simulink model "CubeSatTEST"  (R2024b)
settings: Solver=ode4  StartTime=simul.t0  StopTime=simul.tf  FixedStep=0.01  RelTol=1e-3
values from neighbouring files (symbols this model uses):
  alpha1 = 0.7    [mainSimTEST.m]
  alpha2 = 0.3    [mainSimTEST.m]
undefined symbols (not defined in the file or in its folder): act, DiscIntNeverNeededParam, env, flag, IC, K, orb, sat, sens
libraries: matrix_library x55, simulink_extras x5, simulink x2
(part 1 of 10)
settings Model: SimulationMode=accelerator  Creator=filippocamaleonte  LastModifiedBy=esteb

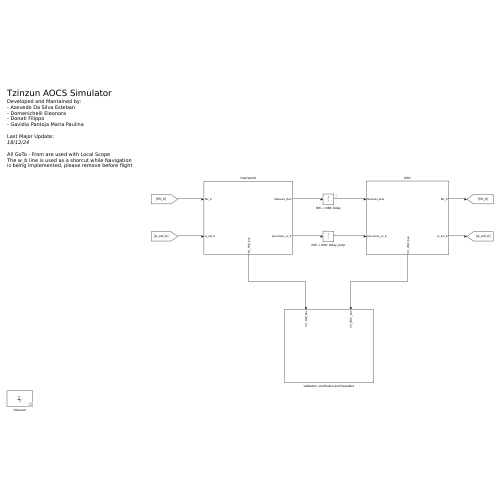
[thumbnail: Simulink's stored preview of the top-level diagram]
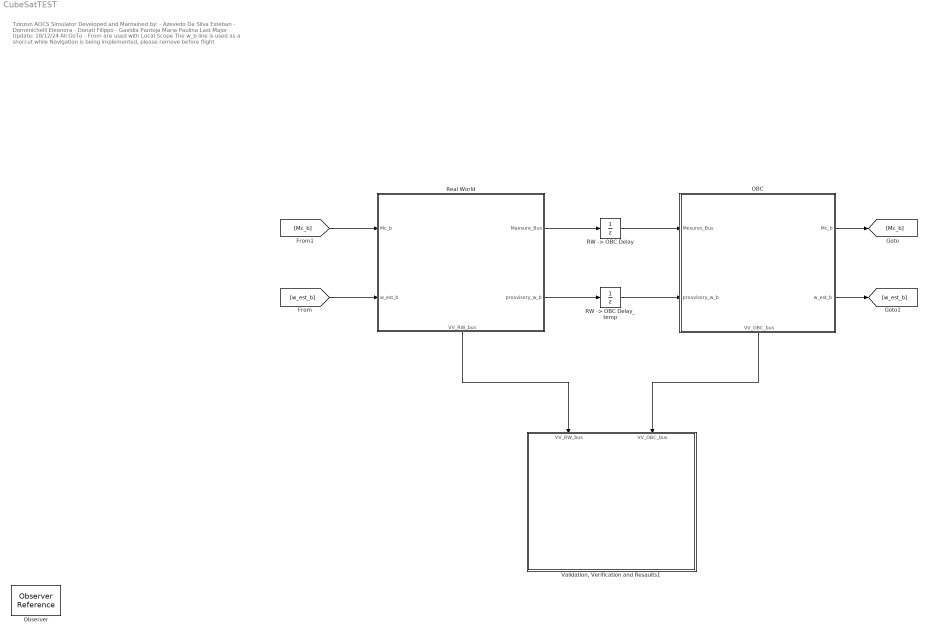
== system CubeSatTEST ==
  note: Tzinzun AOCS Simulator
      | Developed and Mantained by:
      | - Azevedo Da Silva Esteban
      | - Domenichelli Eleonora
      | - Donati Filippo
      | - Gavidia Pantoja Maria Paulina
      |
      | Last Major Update:
      | 18/12/24
      |
      | All GoTo - From are used with Local Scope
      | The w_b line is used as a shorcut while Navigation
      | is being implemented, please remove before flight
  OBC : Subsystem
      settings: PortSchema="{\"entries\":[{\"content\":{\"sides\":[{\"content\":{\"connectorIds\":[\"In1\",\"In2\"]},\"type\":\"ConnectorPlacement.EquallySpacedRectSide\",\"uuid\":\"5088e392-5ef7-43b6-88d2-94fca0031a95\"},{\"content\":{\"connectorIds\":[\"Out1\",\"Out2\"],\"side\":\"RIGHT\"},\"type\":\"ConnectorPlacement.EquallySpacedRectSide\",\"uuid\":\"65d4d952-0f33-4543-97b8-224d6cd7f4c9\"},{\"content\":{\"side\":\"TOP\"},\"type\":\"ConnectorPlacement.EquallySpacedRectSide\",\"uuid\":\"12d55989-2730-40a6-ad18-b5eef3f3e17c\"},{\"content\":{\"connectorIds\":[\"Out3\"],\"side\":\"BOTTOM\"},\"type\":\"ConnectorPlacement.EquallySpacedRectSide\",\"uuid\":\"b2ac3f7e-b4bc-4fee-b426-70088d5715ce\"}]},\"type\":\"ConnectorPlacement.EquallySpacedConnector\",\"uuid\":\"5ce4181d-1e4d-45af-a45d-0aab98c9a049\"}],\"packageUris\":[\"http://schema.mathworks.com/mf0/Connector/R2020b\"],\"version\":\"1.0\"}"
  Observer : ObserverReference  ObserverModelName=CubeSatTEST_Observer1
  "RW -> OBC Delay" : UnitDelay  SampleTime=-1  HasFrameUpgradeWarning=on
  "RW -> OBC Delay_temp" : UnitDelay  SampleTime=-1  HasFrameUpgradeWarning=on
  Real World : Subsystem
      settings: PortSchema="{\"entries\":[{\"content\":{\"sides\":[{\"content\":{\"connectorIds\":[\"In1\",\"In2\"]},\"type\":\"ConnectorPlacement.EquallySpacedRectSide\",\"uuid\":\"5088e392-5ef7-43b6-88d2-94fca0031a95\"},{\"content\":{\"connectorIds\":[\"Out1\",\"Out2\"],\"side\":\"RIGHT\"},\"type\":\"ConnectorPlacement.EquallySpacedRectSide\",\"uuid\":\"65d4d952-0f33-4543-97b8-224d6cd7f4c9\"},{\"content\":{\"side\":\"TOP\"},\"type\":\"ConnectorPlacement.EquallySpacedRectSide\",\"uuid\":\"12d55989-2730-40a6-ad18-b5eef3f3e17c\"},{\"content\":{\"connectorIds\":[\"Out3\"],\"side\":\"BOTTOM\"},\"type\":\"ConnectorPlacement.EquallySpacedRectSide\",\"uuid\":\"7663cd77-36b9-4bef-bf83-4a7645a31ac2\"}]},\"type\":\"ConnectorPlacement.EquallySpacedConnector\",\"uuid\":\"5ce4181d-1e4d-45af-a45d-0aab98c9a049\"}],\"packageUris\":[\"http://schema.mathworks.com/mf0/Connector/R2020b\"],\"version\":\"1.0\"}"
  "Validation, Verification and Resaults1" : Subsystem
      settings: PortSchema="{\"entries\":[{\"content\":{\"sides\":[{\"content\":{},\"type\":\"ConnectorPlacement.EquallySpacedRectSide\",\"uuid\":\"d45fcb8c-a235-4865-973e-7db5dcb51bcf\"},{\"content\":{\"side\":\"RIGHT\"},\"type\":\"ConnectorPlacement.EquallySpacedRectSide\",\"uuid\":\"9c15b117-012a-46d2-951b-db48579a79bd\"},{\"content\":{\"connectorIds\":[\"In1\",\"In2\"],\"side\":\"TOP\"},\"type\":\"ConnectorPlacement.EquallySpacedRectSide\",\"uuid\":\"1325b1ed-c27a-4991-9f5e-80ff75ccfdea\"}]},\"type\":\"ConnectorPlacement.EquallySpacedConnector\",\"uuid\":\"1e5575a1-9967-4d6e-86c8-655c2f02c91c\"}],\"packageUris\":[\"http://schema.mathworks.com/mf0/Connector/R2020b\"],\"version\":\"1.0\"}"
  wires:
  OBC/1(Mc_b) -> [Mc_b]
  "RW -> OBC Delay_temp"/1 -> OBC/2(provvisory_w_b)
  Real World/1(Maesure_Bus) -> "RW -> OBC Delay"/1
  [w_est_b] -> Real World/2(w_est_b)
  Real World/2(provvisory_w_b) -> "RW -> OBC Delay_temp"/1
  Real World/3(VV_RW_bus) -> "Validation, Verification and Resaults1"/1(VV_RW_bus)
  "RW -> OBC Delay"/1 -> OBC/1(Mesures_Bus)
  OBC/3(VV_OBC_bus) -> "Validation, Verification and Resaults1"/2(VV_OBC_bus)
  OBC/2(w_est_b) -> [w_est_b]
  [Mc_b] -> Real World/1(Mc_b)

== system CubeSatTEST/OBC ==
  Mesures_Bus : Inport
  provvisory_w_b : Inport  Port=2
  Bus Selector : BusSelector  OutputSignals=S_meas_b,B_meas_b
  Constant : Constant  Value=alpha1
  Constant1 : Constant  Value=alpha2
  Control : Subsystem
      settings: PortSchema="{\"entries\":[{\"content\":{\"sides\":[{\"content\":{},\"type\":\"ConnectorPlacement.EquallySpacedRectSide\",\"uuid\":\"c22aaece-5395-4ae9-8ea4-e2d3a5a04f7c\"},{\"content\":{\"connectorIds\":[\"Out1\"],\"side\":\"RIGHT\"},\"type\":\"ConnectorPlacement.EquallySpacedRectSide\",\"uuid\":\"8f9c43a1-9386-4a19-ab51-ed4afd641481\"},{\"content\":{\"side\":\"TOP\"},\"type\":\"ConnectorPlacement.EquallySpacedRectSide\",\"uuid\":\"d5c27e22-1cc1-4e6e-857d-4b6af8913d67\"},{\"content\":{\"connectorIds\":[\"In1\",\"In2\"],\"side\":\"BOTTOM\"},\"type\":\"ConnectorPlacement.EquallySpacedRectSide\",\"uuid\":\"f2815a08-d3fb-4840-8d8a-7e5f8666a120\"}]},\"type\":\"ConnectorPlacement.EquallySpacedConnector\",\"uuid\":\"6d356f8e-d841-4478-acc7-b1e45aa749d8\"}],\"packageUris\":[\"http://schema.mathworks.com/mf0/Connector/R2020b\"],\"version\":\"1.0\"}"
  Cos : Trigonometry  Operator=cos
  Discrete-Time Integrator : DiscreteIntegrator  SampleTime=-1  ICPrevOutput=DiscIntNeverNeededParam  ICPrevScaledInput=DiscIntNeverNeededParam
  Dot Product : DotProduct  OutDataTypeStr=Inherit: Inherit via internal rule
  Guidance : Subsystem
  Navigation1 : Subsystem
  Normaliser (with Built In safety) : Subsystem
  Normaliser (with Built In safety)1 : Subsystem
  Reference : Subsystem
  Scope : Scope
  Scope1 : Scope
  Scope2 : Scope  NumInputPorts=3
  Mc_b : Outport
  w_est_b : Outport  Port=2
  VV_OBC_bus : Outport  Port=3
  wires:
  Control/1(Mc_b) -> [Mc_b]
  provvisory_w_b/1 -> Control/2(provvisory_w_b), Scope1/1
  Constant1/1 -> Navigation1/2(alpha2)
  [B_meas_b] -> Navigation1/6(B_b)
  Normaliser (with Built In safety)/1(Out1) -> Navigation1/4(B_N)
  [S_meas_b] -> Navigation1/5(S_b)
  Constant/1 -> Navigation1/1(alpha1)
  Reference/3(B_n) -> Normaliser (with Built In safety)/1(Vector)
  Reference/2(S_n) -> Navigation1/3(S_N)
  Mesures_Bus/1 -> Bus Selector/1, Control/1(Mesures_Bus)
  Bus Selector/1 -> Scope2/2, [S_meas_b], Dot Product/2  "<S_meas_b>"
  Bus Selector/2 -> Normaliser (with Built In safety)1/1(Vector)  "<B_meas_b>"
  Normaliser (with Built In safety)1/1(Out1) -> Dot Product/1, Scope2/1, [B_meas_b]
  Navigation1/1(w_estimated) -> Scope/1
  [Mc_b] -> Mc_b/1
  Cos/1 -> Scope2/3
  Dot Product/1 -> Cos/1

== system CubeSatTEST/Real World ==
  note: Output Interface
  note: Input Interface
  Mc_b : Inport
  w_est_b : Inport  Port=2
  DKE (Dynamics Kinematics Environment) : Subsystem
  Hardware Models : Subsystem
  Scope : Scope
  Maesure_Bus : Outport
  provvisory_w_b : Outport  Port=2
  VV_RW_bus : Outport  Port=3
  wires:
  Hardware Models/2(Measure_Bus) -> [Measure_Bus]
  [Measure_Bus] -> Maesure_Bus/1
  Mc_b/1 -> [Mc_b]
  w_est_b/1 -> [w_est_b]
  Hardware Models/1(Control_Torque_Real) -> [Control_Torque]
  [Control_Torque] -> DKE (Dynamics Kinematics Environment)/1(Control_Torque)
  [Mc_b] -> Hardware Models/4(Mc_b)
  [w_est_b] -> Hardware Models/6(w_est_b)
  DKE (Dynamics Kinematics Environment)/1(w_b) -> Scope/1, provvisory_w_b/1, [w_b]
  DKE (Dynamics Kinematics Environment)/4(B_b) -> [B_b]
  DKE (Dynamics Kinematics Environment)/3(Eclipse) -> [Eclipse]
  DKE (Dynamics Kinematics Environment)/2(S_b) -> [S_b]
  [w_b] -> Hardware Models/5(w_b)
  [S_b] -> Hardware Models/1(S_b)
  [Eclipse] -> Hardware Models/2(Eclipse)
  [B_b] -> Hardware Models/3(B_b)
  Hardware Models/3(vv_Hw_bus) -> [vv_Hw_bus]
  [vv_Hw_bus] -> VV_RW_bus/1

== system CubeSatTEST/Validation, Verification and Resaults1 ==
  VV_RW_bus : Inport
  VV_OBC_bus : Inport  Port=2
  Bus Selector : BusSelector  OutputSignals=sensor_bus.Measure_bus.S_meas_b,sensor_bus.Sun_sensors.Fine_SS,sensor_bus.Sun_sensors.Co1_SS,sensor_bus.Sun_sensors.Co2_SS,sensor_bus.Sun_sensors.Co3_SS,sensor_bus.Sun_sensors.Co4_SS
  Scope : Scope  NumInputPorts=5
  wires:
  VV_RW_bus/1 -> Bus Selector/1
  Bus Selector/6 -> Scope/5  "<Co4_SS>"
  Bus Selector/5 -> Scope/3  "<Co3_SS>"
  Bus Selector/4 -> Scope/4  "<Co2_SS>"
  Bus Selector/3 -> Scope/1  "<Co1_SS>"
  Bus Selector/2 -> Scope/2  "<Fine_SS>"

== system CubeSatTEST/OBC/Control ==
  Mesures_Bus : Inport
  provvisory_w_b : Inport  Port=2
  Acos : Trigonometry  Operator=acos
  Bus Selector : BusSelector  OutputSignals=S_meas_b
  Constant : Constant  Value=0.01
  Constant1 : Constant  Value=[0; 0; 1]
  Demux : Demux  Outputs=3
  Demux1 : Demux  Outputs=3
  Dot Product : DotProduct  OutDataTypeStr=Inherit: Inherit via internal rule
  Mux : Mux  Inputs=3
  Mux1 : Mux  Inputs=5
  Pointing First I : Subsystem
  Radians to Degrees : simulink_extras/Transformations/Radians to Degrees
  Saturation : Saturate  UpperLimit=9e-3  LowerLimit=-9e-3
  Scope : Scope
  Scope1 : Scope
  Selector : Selector  NumberOfDimensions=2  InputPortWidth=3  IndexOptions=Index vector (dialog),Index vector (dialog)  Indices=2,3  OutputSizes=1,1
  Selector1 : Selector  NumberOfDimensions=2  InputPortWidth=3  IndexOptions=Index vector (dialog),Index vector (dialog)  Indices=1,2  OutputSizes=1,1
  Selector2 : Selector  NumberOfDimensions=2  InputPortWidth=3  IndexOptions=Index vector (dialog),Index vector (dialog)  Indices=1,3  OutputSizes=1,1
  Skeleton of Linear Pointing : Subsystem
  Subtract : Sum  Inputs=+-
  Terminator : Terminator
  Test Detumbling : Subsystem
  Mc_b : Outport
  wires:
  Selector1/1 -> Mux/3
  Selector/1 -> Mux/1
  Mux/1 -> Skeleton of Linear Pointing/1(In1)
  Selector2/1 -> Mux/2
  ? -> Selector1/1, Selector/1, Selector2/1
  Mesures_Bus/1 -> Bus Selector/1
  provvisory_w_b/1 -> Demux/1, Test Detumbling/1(w)
  Mux1/1 -> Pointing First I/1(In1)
  Subtract/1 -> Mux1/5
  Demux/3 -> Subtract/1
  Demux/2 -> Mux1/4
  Demux/1 -> Mux1/3
  Bus Selector/1 -> Dot Product/1, Demux1/1  "<S_meas_b>"
  Demux1/1 -> Mux1/1
  Demux1/2 -> Mux1/2
  Pointing First I/1(Mc_b) -> Scope1/1, Saturation/1
  Demux1/3 -> Terminator/1
  Dot Product/1 -> Acos/1
  Radians to Degrees/1 -> Scope/1
  Constant1/1 -> Dot Product/2
  Acos/1 -> Radians to Degrees/1
  Constant/1 -> Subtract/2
  Saturation/1 -> Mc_b/1

== system CubeSatTEST/OBC/Guidance ==
  In1 : Inport
  Sun Pointing Guidance : Subsystem  Commented=on
  Out1 : Outport
  wires:
  In1/1 -> Out1/1

== system CubeSatTEST/OBC/Navigation1 ==
  alpha1 : Inport
  alpha2 : Inport  Port=2
  S_N : Inport  Port=3
  B_N : Inport  Port=4
  S_b : Inport  Port=5
  B_b : Inport  Port=6
  Angular Velocity Extimator : Subsystem  Commented=on
  Angular velocity (w) computing : Subsystem  Commented=on
  Angular velocity (w) computing1 : Subsystem  Commented=on
  DCM TO W : Subsystem
  Demux : Demux  Outputs=3
  Demux1 : Demux  Outputs=3
  MATLAB Function : MATLAB Function  TreatAsAtomicUnit=on
  Mux : Mux  Inputs=3
  Mux1 : Mux  Inputs=3
  Normaliser (with Built In safety)1 : Subsystem
  Normaliser (with Built In safety)2 : Subsystem
  Q method : Subsystem  Commented=on
      settings: PortSchema="{\"entries\":[{\"content\":{\"sides\":[{\"content\":{\"connectorIds\":[\"In1\",\"In2\",\"In3\",\"In4\"]},\"type\":\"ConnectorPlacement.EquallySpacedRectSide\",\"uuid\":\"15956c10-3c30-4cb4-a63c-f434daa5cd48\"},{\"content\":{\"connectorIds\":[\"Out1\"],\"side\":\"RIGHT\"},\"type\":\"ConnectorPlacement.EquallySpacedRectSide\",\"uuid\":\"3f26d307-35c8-43a0-9998-86e1286678fb\"},{\"content\":{\"connectorIds\":[\"In5\",\"In6\"],\"side\":\"TOP\"},\"type\":\"ConnectorPlacement.EquallySpacedRectSide\",\"uuid\":\"55f51305-766e-4e3f-8617-95c7676083b2\"}]},\"type\":\"ConnectorPlacement.EquallySpacedConnector\",\"uuid\":\"09b6cbb7-0430-4316-92af-7ec4423129aa\"}],\"packageUris\":[\"http://schema.mathworks.com/mf0/Connector/R2020b\"],\"version\":\"1.0\"}"
  Scope6 : Scope
  Sequential Rotations : Subsystem  Commented=on
      settings: PortSchema="{\"entries\":[{\"content\":{\"sides\":[{\"content\":{\"connectorIds\":[\"In1\",\"In2\",\"In3\",\"In4\"]},\"type\":\"ConnectorPlacement.EquallySpacedRectSide\",\"uuid\":\"3f30624c-d536-4f4c-9d68-113e77fd2a08\"},{\"content\":{\"connectorIds\":[\"Out1\"],\"side\":\"RIGHT\"},\"type\":\"ConnectorPlacement.EquallySpacedRectSide\",\"uuid\":\"85926a76-b1eb-4ce1-a53a-bd68fe929dfe\"},{\"content\":{\"connectorIds\":[\"In5\",\"In6\"],\"side\":\"TOP\"},\"type\":\"ConnectorPlacement.EquallySpacedRectSide\",\"uuid\":\"d13a957f-b6df-4418-85b8-21ecd6b95f81\"}]},\"type\":\"ConnectorPlacement.EquallySpacedConnector\",\"uuid\":\"e3080881-b5e2-4e0e-904d-d18738ceffcf\"}],\"packageUris\":[\"http://schema.mathworks.com/mf0/Connector/R2020b\"],\"version\":\"1.0\"}"
  Sequential Rotations + Q method : Subsystem
      settings: PortSchema="{\"entries\":[{\"content\":{\"sides\":[{\"content\":{\"connectorIds\":[\"In1\",\"In2\",\"In3\",\"In4\"]},\"type\":\"ConnectorPlacement.EquallySpacedRectSide\",\"uuid\":\"3f30624c-d536-4f4c-9d68-113e77fd2a08\"},{\"content\":{\"connectorIds\":[\"Out1\"],\"side\":\"RIGHT\"},\"type\":\"ConnectorPlacement.EquallySpacedRectSide\",\"uuid\":\"85926a76-b1eb-4ce1-a53a-bd68fe929dfe\"},{\"content\":{\"connectorIds\":[\"In5\",\"In6\"],\"side\":\"TOP\"},\"type\":\"ConnectorPlacement.EquallySpacedRectSide\",\"uuid\":\"d13a957f-b6df-4418-85b8-21ecd6b95f81\"}]},\"type\":\"ConnectorPlacement.EquallySpacedConnector\",\"uuid\":\"e3080881-b5e2-4e0e-904d-d18738ceffcf\"}],\"packageUris\":[\"http://schema.mathworks.com/mf0/Connector/R2020b\"],\"version\":\"1.0\"}"
  Sequential Rotations Playground : Subsystem  Commented=on
  Transfer Fcn1 : TransferFcn  Denominator=[50 1]
  Transfer Fcn2 : TransferFcn  Denominator=[10 1]
  Transfer Fcn3 : TransferFcn  Denominator=[50 1]
  Transfer Fcn4 : TransferFcn  Denominator=[50 1]
  Transfer Fcn5 : TransferFcn  Denominator=[10 1]
  Transfer Fcn6 : TransferFcn  Denominator=[10 1]
  w_estimated : Outport
  wires:
  alpha1/1 -> Sequential Rotations + Q method/5(alpha 1)
  alpha2/1 -> Sequential Rotations + Q method/6(alpha 2)
  MATLAB Function/1(DCM) -> Scope6/1, DCM TO W/1(A(B/N))
  DCM TO W/1(w) -> w_estimated/1
  Angular velocity (w) computing1/1(w_estimated) -> ?
  Sequential Rotations + Q method/1(q_estimated) -> MATLAB Function/1(q)
  S_b/1 -> Demux/1
  Demux/1 -> Transfer Fcn1/1
  Demux/2 -> Transfer Fcn3/1
  Demux/3 -> Transfer Fcn4/1
  Transfer Fcn3/1 -> Mux/2
  Transfer Fcn1/1 -> Mux/1
  Transfer Fcn4/1 -> Mux/3
  S_N/1 -> Sequential Rotations + Q method/2(Sn)
  Demux1/2 -> Transfer Fcn5/1
  Transfer Fcn6/1 -> Mux1/3
  Transfer Fcn2/1 -> Mux1/1
  Demux1/3 -> Transfer Fcn6/1
  Transfer Fcn5/1 -> Mux1/2
  Demux1/1 -> Transfer Fcn2/1
  B_N/1 -> Sequential Rotations + Q method/4(Bn)
  B_b/1 -> Demux1/1
  Mux1/1 -> Normaliser (with Built In safety)2/1(Vector)
  Mux/1 -> Normaliser (with Built In safety)1/1(Vector)
  Normaliser (with Built In safety)1/1(Out1) -> Sequential Rotations + Q method/1(S_b)
  Normaliser (with Built In safety)2/1(Out1) -> Sequential Rotations + Q method/3(B_b)

== system CubeSatTEST/OBC/Normaliser (with Built In safety) ==
  Vector : Inport
  Constant : Constant  Value=[0; 0; 0]  VectorParams1D=off
  Norm1 : Subsystem
  Protected Division : Subsystem
  Switch : Switch  Criteria=u2 ~= 0  SaturateOnIntegerOverflow=off  InputSameDT=off
  Out1 : Outport
  wires:
  Norm1/1(Norm) -> Switch/2, Protected Division/2(Norm)  "norm_r"
  Switch/1 -> Out1/1
  Protected Division/1(Out1) -> Switch/1
  Vector/1 -> Protected Division/1(Vector), Norm1/1(Vector)
  Constant/1 -> Switch/3

== system CubeSatTEST/OBC/Normaliser (with Built In safety)1 ==
  Vector : Inport
  Constant : Constant  Value=[0; 0; 0]  VectorParams1D=off
  Norm1 : Subsystem
  Protected Division : Subsystem
  Switch : Switch  Criteria=u2 ~= 0  SaturateOnIntegerOverflow=off  InputSameDT=off
  Out1 : Outport
  wires:
  Norm1/1(Norm) -> Switch/2, Protected Division/2(Norm)  "norm_r"
  Switch/1 -> Out1/1
  Protected Division/1(Out1) -> Switch/1
  Vector/1 -> Protected Division/1(Vector), Norm1/1(Vector)
  Constant/1 -> Switch/3

== system CubeSatTEST/OBC/Reference ==
  Conical Shadow Model : Subsystem
  Constant1 : Constant  Value=orb.i
  Kepler Integrator1 : Subsystem
  LVLH Evolution wtr of Earth2 : Subsystem
  Magnetic Field order 1 : Subsystem
  SpaceCraft position wrt ECI1 : Subsystem
  Sun Direction Circular Orbit : Subsystem
  A_ln : Outport
  S_n : Outport  Port=2
  B_n : Outport  Port=3
  r_n : Outport  Port=4
  eclipseFlag : Outport  Port=5
  wires:
  Constant1/1 -> LVLH Evolution wtr of Earth2/2(i)
  LVLH Evolution wtr of Earth2/1(A_ln) -> A_ln/1
  Sun Direction Circular Orbit/1(S_n) -> S_n/1, Conical Shadow Model/1(S_n)
  SpaceCraft position wrt ECI1/1(r_n) -> Magnetic Field order 1/1(Vector), r_n/1, Conical Shadow Model/2(r_n)
  Conical Shadow Model/1(eclipseFlag) -> eclipseFlag/1
  Magnetic Field order 1/1(B_n) -> B_n/1
  Kepler Integrator1/2(OM) -> SpaceCraft position wrt ECI1/2(OM), LVLH Evolution wtr of Earth2/3(OM)
  Kepler Integrator1/1(th) -> SpaceCraft position wrt ECI1/1(th), LVLH Evolution wtr of Earth2/1(th)

== system CubeSatTEST/Real World/DKE (Dynamics Kinematics Environment) ==
  note: Input Interface
  note: Input Interface
  Control_Torque : Inport
  Acos : Trigonometry  Operator=acos
  Acos1 : Trigonometry  Operator=acos
  Constant1 : Constant  Value=[0; 0; -1]
  Constant2 : Constant  Value=[0; 0; 1]
  Dot Product : DotProduct  OutDataTypeStr=Inherit: Inherit via internal rule
  Dot Product1 : DotProduct  OutDataTypeStr=Inherit: Inherit via internal rule
  Dynamics : Subsystem
  Environment : Subsystem
  Kinematics : Subsystem
  Radians to Degrees : simulink_extras/Transformations/Radians to Degrees
  Radians to Degrees1 : simulink_extras/Transformations/Radians to Degrees
  Scope : Scope
  Scope1 : Scope
  Scope2 : Scope
  Sum : Sum  Inputs=|++
  To Workspace : ToWorkspace  VariableName=eclipse  SampleTime=-1
  w_b : Outport
  S_b : Outport  Port=2
  Eclipse : Outport  Port=3
  B_b : Outport  Port=4
  wires:
  Dynamics/1(w_b) -> [w_b], Kinematics/1(w_b)
  Sum/1 -> Dynamics/1(M_ext)
  Environment/4(Disturbance_torque) -> Sum/2
  [w_b] -> w_b/1
  Kinematics/3(r_n) -> Environment/3(r_n)
  Kinematics/1(A_bn) -> Scope2/1, Environment/1(A_bn)
  Kinematics/2(A_bl) -> Environment/2(A_bl)
  Control_Torque/1 -> [Control_Torque]
  [S_b] -> S_b/1
  [eclipse] -> Eclipse/1
  [B_b] -> B_b/1
  Environment/1(Eclipse) -> To Workspace/1, [eclipse]
  Environment/3(B_b) -> [B_b]
  [Control_Torque] -> Sum/1
  Radians to Degrees/1 -> Scope/1
  Dot Product/1 -> Acos/1
  Constant1/1 -> Dot Product/2
  Acos/1 -> Radians to Degrees/1
  Radians to Degrees1/1 -> Scope1/1
  Dot Product1/1 -> Acos1/1
  Constant2/1 -> Dot Product1/2
  Acos1/1 -> Radians to Degrees1/1
  Environment/2(S_b) -> Dot Product1/1, [S_b]

== system CubeSatTEST/Real World/Hardware Models ==
  note: Hardware Models
  note: Input Interface
  note: Output Interface
  S_b : Inport
  Eclipse : Inport  Port=2
  B_b : Inport  Port=3
  Mc_b : Inport  Port=4
  w_b : Inport  Port=5
  w_est_b : Inport  Port=6
  Actuators : Subsystem
  Bus Creator : BusCreator  Inputs=2
  Sensors : Subsystem
  Control_Torque_Real : Outport
  Measure_Bus : Outport  Port=2
  vv_Hw_bus : Outport  Port=3
  wires:
  Sensors/1(Measure) -> [measure_bus]
  [measure_bus] -> Measure_Bus/1
  [S_b] -> Sensors/1(S_b)
  [control_torque] -> Control_Torque_Real/1
  Actuators/1(Control_Torque_b) -> [control_torque]
  [eclipse] -> Sensors/2(Eclipse)
  S_b/1 -> [S_b]
  Eclipse/1 -> [eclipse]
  B_b/1 -> [B_b]
  w_est_b/1 -> [w_est_b]
  w_b/1 -> [w_b]
  Mc_b/1 -> [Mc_b]
  [B_b] -> Sensors/3(B_b)
  [w_est_b] -> Actuators/2(w_est_b)
  [w_b] -> Actuators/3(w_b)
  [Mc_b] -> Actuators/1(Mc_b)
  Sensors/2(vv_Sensor_bus) -> [vv_Sensor_bus]
  Actuators/2(vv_act_bus) -> [vv_act_bus]
  [vv_Sensor_bus] -> Bus Creator/1
  [vv_act_bus] -> Bus Creator/2
  Bus Creator/1 -> vv_Hw_bus/1

== system CubeSatTEST/OBC/Control/Pointing First I ==
  In1 : Inport
  Constant : Constant  Value=K
  Gain : Gain  Gain=-1
  MatrixMultiply : Product  Multiplication=Matrix(*)
  Mc_b : Outport
  wires:
  MatrixMultiply/1 -> Mc_b/1
  In1/1 -> MatrixMultiply/2
  Constant/1 -> Gain/1
  Gain/1 -> MatrixMultiply/1

== system CubeSatTEST/OBC/Control/Skeleton of Linear Pointing ==
  In1 : Inport
  w : Inport  Port=2
  Add : Sum
  Constant : Constant  Value=0
  Demux : Demux  Outputs=3
  Demux1 : Demux  Outputs=3
  Gain : Gain  Gain=-4.086e-5
  Gain1 : Gain  Gain=-8.9519e-5
  Gain2 : Gain  Gain=-0.0021
  Gain3 : Gain  Gain=-0.0047
  Gain4 : Gain  Gain=-0.0025
  Mux : Mux  Inputs=3
  Mux1 : Mux  Inputs=3
  Terminator : Terminator
  Mc : Outport
  wires:
  Demux/3 -> Terminator/1
  In1/1 -> Demux/1
  w/1 -> Demux1/1
  Constant/1 -> Mux/3
  Gain/1 -> Mux/1
  Demux/1 -> Gain/1
  Demux/2 -> Gain1/1
  Gain1/1 -> Mux/2
  Demux1/1 -> Gain2/1
  Gain2/1 -> Mux1/1
  Demux1/3 -> Gain4/1
  Gain4/1 -> Mux1/3
  Gain3/1 -> Mux1/2
  Demux1/2 -> Gain3/1
  Mux/1 -> Add/1
  Add/1 -> Mc/1
  Mux1/1 -> Add/2

== system CubeSatTEST/OBC/Control/Test Detumbling ==
  w : Inport
  Constant : Constant  Value=[[-0.03, 0, 0]; [0, -0.003, 0]; [0, 0, -0.003]]
  Constant1 : Constant  Value=[0; 0; 0]
  Gain : Gain  Commented=through  Gain=5e5
  Matrix Multiply : Product  Multiplication=Matrix(*)
  Scope : Scope
  Subtract : Sum  Inputs=+-
  Mc : Outport
  wires:
  Subtract/1 -> Matrix Multiply/2
  Constant1/1 -> Subtract/2
  Matrix Multiply/1 -> Mc/1
  Constant/1 -> Gain/1
  w/1 -> Scope/1, Subtract/1
  Gain/1 -> Matrix Multiply/1

== system CubeSatTEST/OBC/Guidance/Sun Pointing Guidance ==
  In1 : Inport
  Attitude Error : Subsystem
  Pointing quaternion (1dof) : Subsystem
  Out1 : Outport
  wires:
  In1/1 -> Out1/1
  Pointing quaternion (1dof)/1(qc) -> Attitude Error/1(qc)

== system CubeSatTEST/OBC/Navigation1/Angular Velocity Extimator ==
  q_estimated : Inport
  Demux : Demux
  Discrete Derivative : simulink/Discrete/Discrete Derivative  gainval=1.0  ICPrevScaledInput=0.0  OutMin=[]  OutMax=[]  OutDataType=fixdt(1, 16)  OutScaling=2^-10  DoSatur=off
  Gain : Gain  Gain=2
  MatrixMultiply : Product  Multiplication=Matrix(*)
  Mux : Mux
  Transfer Fcn{1..4} (4 alike) : TransferFcn  Denominator=[50 1]
  Transpose : Math  Operator=transpose
  Xi(q) : Subsystem
  Out1 : Outport
  wires:
  q_estimated/1 -> Demux/1, Xi(q)/1(In1)
  Xi(q)/1(Out1) -> Transpose/1
  Discrete Derivative/1 -> MatrixMultiply/2
  Transpose/1 -> Gain/1
  Gain/1 -> MatrixMultiply/1
  MatrixMultiply/1 -> Out1/1
  Mux/1 -> Discrete Derivative/1
  Demux/4 -> Transfer Fcn4/1
  Demux/1 -> Transfer Fcn1/1
  Demux/3 -> Transfer Fcn3/1
  Demux/2 -> Transfer Fcn2/1
  Transfer Fcn2/1 -> Mux/2
  Transfer Fcn1/1 -> Mux/1
  Transfer Fcn3/1 -> Mux/3
  Transfer Fcn4/1 -> Mux/4

== system CubeSatTEST/OBC/Navigation1/Angular velocity (w) computing ==
  q_estimated : Inport
  Constant : Constant  Value=2
  Demux : Demux
  Derivative{,1..3} (4 alike) : Derivative
  Matrix Multiply : Product  Multiplication=Matrix(*)
  Mux : Mux
  Product : Product
  Q(q) : Subsystem
  Transfer Fcn : TransferFcn  Numerator=1  Denominator=[3 1]
  Transfer Fcn1 : TransferFcn  Denominator=[3 1]
  Transfer Fcn2 : TransferFcn  Denominator=[3 1]
  Transfer Fcn3 : TransferFcn  Denominator=[3 1]
  w_estimated : Outport
  wires:
  q_estimated/1 -> [q]
  [q] -> Demux/1
  Demux/1 -> Derivative/1
  Demux/2 -> Derivative1/1
  Demux/3 -> Derivative2/1
  Demux/4 -> Derivative3/1
  [q] -> Q(q)/1(q)
  Mux/1 -> [q_dot]
  [Q] -> Product/2
  Constant/1 -> Product/1
  [q_dot] -> Matrix Multiply/2
  Derivative/1 -> Transfer Fcn3/1
  Derivative1/1 -> Transfer Fcn2/1
  Derivative2/1 -> Transfer Fcn1/1
  Derivative3/1 -> Transfer Fcn/1
  Product/1 -> Matrix Multiply/1
  Q(q)/1(Ksi(q)) -> [Q]
  Matrix Multiply/1 -> w_estimated/1
  Transfer Fcn3/1 -> Mux/1
  Transfer Fcn2/1 -> Mux/2
  Transfer Fcn1/1 -> Mux/3
  Transfer Fcn/1 -> Mux/4

== system CubeSatTEST/OBC/Navigation1/Angular velocity (w) computing1 ==
  q_estimated : Inport
  Constant : Constant  Value=2
  Demux1 : Demux
  Demux2 : Demux
  Derivative{4..7} (4 alike) : Derivative
  Matrix Multiply : Product  Multiplication=Matrix(*)
  Mux1 : Mux
  Product : Product
  Q(q) computing : Subsystem
  Transfer Fcn : TransferFcn  Commented=through  Numerator=1  Denominator=[15 1]
  Transfer Fcn1 : TransferFcn  Commented=through  Denominator=[15 1]
  Transfer Fcn2 : TransferFcn  Commented=through  Denominator=[15 1]
  Transfer Fcn3 : TransferFcn  Commented=through  Denominator=[15 1]
  w_estimated : Outport
  wires:
  q_estimated/1 -> [q]
  [q] -> Demux1/1
  Demux1/1 -> Q(q) computing/1(q1)
  Demux1/4 -> Q(q) computing/4(q4)
  Demux1/3 -> Q(q) computing/3(q3)
  Demux1/2 -> Q(q) computing/2(q2)
  [Q] -> Product/2
  Constant/1 -> Product/1
  [q_dot] -> Matrix Multiply/2
  Matrix Multiply/1 -> w_estimated/1
  Product/1 -> Matrix Multiply/1
  Q(q) computing/1(Q(q)) -> [Q]
  Transfer Fcn2/1 -> Mux1/2
  Derivative7/1 -> Transfer Fcn/1
  Derivative4/1 -> Transfer Fcn3/1
  Transfer Fcn3/1 -> Mux1/1
  Transfer Fcn/1 -> Mux1/4
  Derivative5/1 -> Transfer Fcn2/1
  Demux2/3 -> Derivative6/1
  Demux2/4 -> Derivative7/1
  Mux1/1 -> [q_dot]
  Demux2/2 -> Derivative5/1
  Demux2/1 -> Derivative4/1
  [q] -> Demux2/1
  Transfer Fcn1/1 -> Mux1/3
  Derivative6/1 -> Transfer Fcn1/1

== system CubeSatTEST/OBC/Navigation1/DCM TO W ==
  A(B/N) : Inport
  1 : Selector  NumberOfDimensions=2  InputPortWidth=3  IndexOptions=Index vector (dialog),Index vector (dialog)  Indices=3,2  OutputSizes=1,1
  11 : Selector  NumberOfDimensions=2  InputPortWidth=3  IndexOptions=Index vector (dialog),Index vector (dialog)  Indices=1,1  OutputSizes=1,1
  12 : Selector  NumberOfDimensions=2  InputPortWidth=3  IndexOptions=Index vector (dialog),Index vector (dialog)  Indices=1,2  OutputSizes=1,1
  13 : Selector  NumberOfDimensions=2  InputPortWidth=3  IndexOptions=Index vector (dialog),Index vector (dialog)  Indices=1,3  OutputSizes=1,1
  2 : Selector  NumberOfDimensions=2  InputPortWidth=3  IndexOptions=Index vector (dialog),Index vector (dialog)  Indices=1,3  OutputSizes=1,1
  21 : Selector  NumberOfDimensions=2  InputPortWidth=3  IndexOptions=Index vector (dialog),Index vector (dialog)  Indices=2,1  OutputSizes=1,1
  22 : Selector  NumberOfDimensions=2  InputPortWidth=3  IndexOptions=Index vector (dialog),Index vector (dialog)  Indices=2,2  OutputSizes=1,1
  23 : Selector  NumberOfDimensions=2  InputPortWidth=3  IndexOptions=Index vector (dialog),Index vector (dialog)  Indices=2,3  OutputSizes=1,1
  3 : Selector  NumberOfDimensions=2  InputPortWidth=3  IndexOptions=Index vector (dialog),Index vector (dialog)  Indices=2,1  OutputSizes=1,1
  31 : Selector  NumberOfDimensions=2  InputPortWidth=3  IndexOptions=Index vector (dialog),Index vector (dialog)  Indices=3,1  OutputSizes=1,1
  32 : Selector  NumberOfDimensions=2  InputPortWidth=3  IndexOptions=Index vector (dialog),Index vector (dialog)  Indices=3,2  OutputSizes=1,1
  33 : Selector  NumberOfDimensions=2  InputPortWidth=3  IndexOptions=Index vector (dialog),Index vector (dialog)  Indices=3,3  OutputSizes=1,1
  4 : Selector  NumberOfDimensions=2  InputPortWidth=3  IndexOptions=Index vector (dialog),Index vector (dialog)  Indices=2,3  OutputSizes=1,1
  5 : Selector  NumberOfDimensions=2  InputPortWidth=3  IndexOptions=Index vector (dialog),Index vector (dialog)  Indices=3,1  OutputSizes=1,1
  6 : Selector  NumberOfDimensions=2  InputPortWidth=3  IndexOptions=Index vector (dialog),Index vector (dialog)  Indices=1,2  OutputSizes=1,1
  Add : Sum  Inputs=+-
  Add1 : Sum  Inputs=+-
  Add2 : Sum  Inputs=+-
  Discrete Derivative : simulink/Discrete/Discrete Derivative  gainval=1.0  ICPrevScaledInput=0.0  OutMin=[]  OutMax=[]  OutDataType=fixdt(1, 16)  OutScaling=2^-10  DoSatur=off
  From : From
  From2 : From
  Gain : Gain  Gain=-1
  Gain1 : Gain  Gain=0.5
  Gain2 : Gain  Gain=0.5
  Gain3 : Gain  Gain=0.5
  Goto : Goto
  Matrix Concatenate : Concatenate  NumInputs=3  Mode=Multidimensional array  ConcatenateDimension=2
  Matrix Concatenate1 : Concatenate  NumInputs=3  Mode=Multidimensional array  ConcatenateDimension=2
  Matrix Concatenate2 : Concatenate  NumInputs=3  Mode=Multidimensional array  ConcatenateDimension=2
  Matrix Concatenate3 : Concatenate  NumInputs=3  Mode=Multidimensional array
  Mux : Mux  Inputs=3
  Product : Product  Multiplication=Matrix(*)
  Scope : Scope
  Transfer Fcn{1..9} (9 alike) : TransferFcn  Denominator=[10 1]
  Transpose : matrix_library/Transpose
  w : Outport
  wires:
  A(B/N)/1 -> Goto/1
  From/1 -> 23/1, 31/1, 32/1, 33/1, 22/1, 21/1, 11/1, 12/1, 13/1
  11/1 -> Transfer Fcn1/1
  33/1 -> Transfer Fcn9/1
  32/1 -> Transfer Fcn8/1
  31/1 -> Transfer Fcn7/1
  23/1 -> Transfer Fcn6/1
  22/1 -> Transfer Fcn5/1
  21/1 -> Transfer Fcn4/1
  13/1 -> Transfer Fcn3/1
  12/1 -> Transfer Fcn2/1
  Matrix Concatenate2/1 -> Matrix Concatenate3/3
  Matrix Concatenate1/1 -> Matrix Concatenate3/2
  Matrix Concatenate/1 -> Matrix Concatenate3/1
  Matrix Concatenate3/1 -> Discrete Derivative/1
  Gain/1 -> Product/1
  [dA] -> Gain/1
  Transpose/1 -> Product/2
  From2/1 -> Transpose/1
  Mux/1 -> w/1
  3/1 -> Add2/1
  6/1 -> Add2/2
  Add/1 -> Gain1/1
  Add1/1 -> Gain2/1
  Add2/1 -> Gain3/1
  2/1 -> Add1/1
  5/1 -> Add1/2
  1/1 -> Add/1
  Gain1/1 -> Mux/1
  Gain2/1 -> Mux/2
  Gain3/1 -> Mux/3
  Transfer Fcn1/1 -> Matrix Concatenate/1
  Transfer Fcn2/1 -> Matrix Concatenate/2
  Transfer Fcn3/1 -> Matrix Concatenate/3
  Transfer Fcn4/1 -> Matrix Concatenate1/1
  Transfer Fcn5/1 -> Matrix Concatenate1/2
  Transfer Fcn6/1 -> Matrix Concatenate1/3
  Transfer Fcn7/1 -> Matrix Concatenate2/1
  Transfer Fcn8/1 -> Matrix Concatenate2/2
  Transfer Fcn9/1 -> Matrix Concatenate2/3
  Product/1 -> 5/1, 6/1, 3/1, 4/1, 1/1, 2/1
  4/1 -> Add/2
  Discrete Derivative/1 -> Scope/1, [dA]

== system CubeSatTEST/OBC/Navigation1/Normaliser (with Built In safety)1 ==
  Vector : Inport
  Constant : Constant  Value=[0; 0; 0]  VectorParams1D=off
  Norm1 : Subsystem
  Protected Division : Subsystem
  Switch : Switch  Criteria=u2 ~= 0  SaturateOnIntegerOverflow=off  InputSameDT=off
  Out1 : Outport
  wires:
  Norm1/1(Norm) -> Switch/2, Protected Division/2(Norm)  "norm_r"
  Switch/1 -> Out1/1
  Protected Division/1(Out1) -> Switch/1
  Vector/1 -> Protected Division/1(Vector), Norm1/1(Vector)
  Constant/1 -> Switch/3

== system CubeSatTEST/OBC/Navigation1/Normaliser (with Built In safety)2 ==
  Vector : Inport
  Constant : Constant  Value=[0; 0; 0]  VectorParams1D=off
  Norm1 : Subsystem
  Protected Division : Subsystem
  Switch : Switch  Criteria=u2 ~= 0  SaturateOnIntegerOverflow=off  InputSameDT=off
  Out1 : Outport
  wires:
  Norm1/1(Norm) -> Switch/2, Protected Division/2(Norm)  "norm_r"
  Switch/1 -> Out1/1
  Protected Division/1(Out1) -> Switch/1
  Vector/1 -> Protected Division/1(Vector), Norm1/1(Vector)
  Constant/1 -> Switch/3

== system CubeSatTEST/OBC/Navigation1/Q method ==
  S_b : Inport
  S_N : Inport  Port=2
  B_b : Inport  Port=3
  B_N : Inport  Port=4
  alpha 1 : Inport  Port=5
  alpha 2 : Inport  Port=6
  B computing : Subsystem
      settings: PortSchema="{\"entries\":[{\"content\":{\"sides\":[{\"content\":{\"connectorIds\":[\"In1\",\"In2\",\"In3\",\"In4\"]},\"type\":\"ConnectorPlacement.EquallySpacedRectSide\",\"uuid\":\"50fc9399-82b5-4b10-921b-f93011029ce3\"},{\"content\":{\"connectorIds\":[\"Out1\"],\"side\":\"RIGHT\"},\"type\":\"ConnectorPlacement.EquallySpacedRectSide\",\"uuid\":\"3981c554-ab38-4f62-9b84-94877d1cd2ff\"},{\"content\":{\"connectorIds\":[\"Out2\",\"Out3\"],\"side\":\"TOP\"},\"type\":\"ConnectorPlacement.EquallySpacedRectSide\",\"uuid\":\"ba062d99-6f44-4068-8114-c0cfa81f1ff2\"},{\"content\":{\"connectorIds\":[\"In5\",\"In6\"],\"side\":\"BOTTOM\"},\"type\":\"ConnectorPlacement.EquallySpacedRectSide\",\"uuid\":\"0ce0d8e8-da8b-4b2d-90df-7b0bc851bc5b\"}]},\"type\":\"ConnectorPlacement.EquallySpacedConnector\",\"uuid\":\"bcda7430-c6c8-4f59-a99a-b367d20ffcb5\"}],\"packageUris\":[\"http://schema.mathworks.com/mf0/Connector/R2020b\"],\"version\":\"1.0\"}"
  S and Z matrix computing : Subsystem
  Scope : Scope
  Subsystem : Subsystem
      settings: PortSchema="{\"entries\":[{\"content\":{\"sides\":[{\"content\":{\"connectorIds\":[\"Out1\"]},\"type\":\"ConnectorPlacement.EquallySpacedRectSide\",\"uuid\":\"5768cb62-7f28-4cce-8da1-dcdd14add895\"},{\"content\":{\"side\":\"RIGHT\"},\"type\":\"ConnectorPlacement.EquallySpacedRectSide\",\"uuid\":\"8778aa17-5802-4f6c-9df9-b85455c7c074\"},{\"content\":{\"connectorIds\":[\"In1\",\"In2\"],\"side\":\"TOP\"},\"type\":\"ConnectorPlacement.EquallySpacedRectSide\",\"uuid\":\"8a3cb844-269f-4d3f-b8ee-2af4584390c1\"},{\"content\":{\"connectorIds\":[\"In3\",\"In4\",\"In5\",\"In6\"],\"side\":\"BOTTOM\"},\"type\":\"ConnectorPlacement.EquallySpacedRectSide\",\"uuid\":\"ccc3bad4-265e-44f4-a8b0-aae769a28e60\"}]},\"type\":\"ConnectorPlacement.EquallySpacedConnector\",\"uuid\":\"9389ccda-4d08-49a8-9951-bd9019203c57\"}],\"packageUris\":[\"http://schema.mathworks.com/mf0/Connector/R2020b\"],\"version\":\"1.0\"}"
  q_opt computing : Subsystem
      settings: PortSchema="{\"entries\":[{\"content\":{\"sides\":[{\"content\":{\"connectorIds\":[\"In1\",\"In2\"]},\"type\":\"ConnectorPlacement.EquallySpacedRectSide\",\"uuid\":\"077e0174-8a2c-4f76-bac9-e91df836f5e1\"},{\"content\":{\"connectorIds\":[\"Out1\",\"In4\"],\"side\":\"RIGHT\"},\"type\":\"ConnectorPlacement.EquallySpacedRectSide\",\"uuid\":\"0e923535-8f32-4607-bd4a-42896d211835\"},{\"content\":{\"connectorIds\":[\"In3\"],\"side\":\"TOP\"},\"type\":\"ConnectorPlacement.EquallySpacedRectSide\",\"uuid\":\"91682e2a-1ae8-44b6-9458-d5d75f2c9b10\"},{\"content\":{\"side\":\"BOTTOM\"},\"type\":\"ConnectorPlacement.EquallySpacedRectSide\",\"uuid\":\"ebee2d10-c6a3-420b-a3da-5d4d259a0e4d\"}]},\"type\":\"ConnectorPlacement.EquallySpacedConnector\",\"uuid\":\"6651e596-192f-4f32-9855-13a8c081df01\"}],\"packageUris\":[\"http://schema.mathworks.com/mf0/Connector/R2020b\"],\"version\":\"1.0\"}"
  q_estimated : Outport
  wires:
  alpha 1/1 -> [alpha1]
  [B_b] -> B computing/3(Bb)
  S_b/1 -> [S_b]
  [B_N] -> B computing/4(BN)
  [S_N] -> B computing/2(SN)
  B computing/1(B) -> q_opt computing/4(B), S and Z matrix computing/1(B)
  [S_N] -> Subsystem/6(S_N)
  [B_b] -> Subsystem/3(B_b)
  [S_b] -> Subsystem/5(S_b)
  B_N/1 -> [B_N]
  S_N/1 -> [S_N]
  B_b/1 -> [B_b]
  [alpha1] -> B computing/5(alpha 1)
  [S_b] -> B computing/1(Sb)
  S and Z matrix computing/1(S) -> q_opt computing/1(S)
  [alpha2] -> B computing/6(alpha 2)
  alpha 2/1 -> [alpha2]
  S and Z matrix computing/2(Z) -> q_opt computing/2(Z)
  q_opt computing/1(q_opt) -> q_estimated/1
  [B_N] -> Subsystem/4(B_N)
  B computing/2(alpha1_normalised) -> Subsystem/2(alpha1_normalised)
  B computing/3(alpha2_normalised) -> Subsystem/1(alpha2_normalised)
  Subsystem/1(lambda_max) -> Scope/1, q_opt computing/3(lambda_max)

== system CubeSatTEST/OBC/Navigation1/Sequential Rotations ==
  S_b : Inport
  Sn : Inport  Port=2
  B_b : Inport  Port=3
  Bn : Inport  Port=4
  alpha 1 : Inport  Port=5
  alpha 2 : Inport  Port=6
  Abs : Abs  SaturateOnIntegerOverflow=off
  Abs1 : Abs  SaturateOnIntegerOverflow=off
  If : If  IfExpression=u1 < 0
  If Action Subsystem : Subsystem  TreatAsAtomicUnit=on
  If Action Subsystem1 : Subsystem  TreatAsAtomicUnit=on
  If Action Subsystem2 : Subsystem  TreatAsAtomicUnit=on
  If Action Subsystem3 : Subsystem  TreatAsAtomicUnit=on
  If1 : If  IfExpression=u1 < 0
  Merge : Merge
  Merge1 : Merge
  Merge2 : Merge
  Q method : Subsystem
      settings: PortSchema="{\"entries\":[{\"content\":{\"sides\":[{\"content\":{\"connectorIds\":[\"In1\",\"In2\",\"In3\",\"In4\"]},\"type\":\"ConnectorPlacement.EquallySpacedRectSide\",\"uuid\":\"15956c10-3c30-4cb4-a63c-f434daa5cd48\"},{\"content\":{\"connectorIds\":[\"Out1\"],\"side\":\"RIGHT\"},\"type\":\"ConnectorPlacement.EquallySpacedRectSide\",\"uuid\":\"3f26d307-35c8-43a0-9998-86e1286678fb\"},{\"content\":{\"connectorIds\":[\"In5\",\"In6\"],\"side\":\"TOP\"},\"type\":\"ConnectorPlacement.EquallySpacedRectSide\",\"uuid\":\"55f51305-766e-4e3f-8617-95c7676083b2\"}]},\"type\":\"ConnectorPlacement.EquallySpacedConnector\",\"uuid\":\"09b6cbb7-0430-4316-92af-7ec4423129aa\"}],\"packageUris\":[\"http://schema.mathworks.com/mf0/Connector/R2020b\"],\"version\":\"1.0\"}"
  Relay : Relay  OnSwitchValue=0.5  OffSwitchValue=0.2  OffOutputValue=-1
  Relay1 : Relay  OnSwitchValue=0.5  OffSwitchValue=0.2  OffOutputValue=-1
  Scope : Scope
  Scope2 : Scope  NumInputPorts=2
  Scope3 : Scope  NumInputPorts=2
  Selector : Selector  InputPortWidth=4  IndexOptions=Index vector (dialog)  Indices=4  OutputSizes=1
  Selector1 : Selector  InputPortWidth=4  IndexOptions=Index vector (dialog)  Indices=4  OutputSizes=1
  Unit Delay : UnitDelay  InitialCondition=[0;0;0;1]  SampleTime=-1  HasFrameUpgradeWarning=on
  Out1 : Outport
  wires:
  alpha 2/1 -> Q method/6(alpha 2)
  alpha 1/1 -> Q method/5(alpha 1)
  S_b/1 -> Q method/1(S_b)
  B_b/1 -> Q method/2(B_b)
  Unit Delay/1 -> Scope/1, [flag]
  Selector/1 -> Abs/1
  [flag] -> Selector/1
  Selector1/1 -> Abs1/1
  Abs1/1 -> Scope2/2, Relay1/1
  [flag] -> Selector1/1
  Merge/1 -> Q method/3(S_N)
  Merge1/1 -> Q method/4(B_N)
  If/2 -> If Action Subsystem/Action
  If Action Subsystem/1(Out1) -> Merge/1
  If Action Subsystem/2(Out2) -> Merge1/1
  Sn/1 -> If Action Subsystem2/1(Sn), If Action Subsystem/1(Sn)
  Bn/1 -> If Action Subsystem2/2(Bn), If Action Subsystem/2(Bn)
  If Action Subsystem1/1(Out1) -> Merge2/2
  If1/2 -> If Action Subsystem1/Action
  If/1 -> If Action Subsystem2/Action
  [flag] -> If Action Subsystem2/3(flag)
  If Action Subsystem2/1(S_n') -> Merge/2
  If Action Subsystem2/2(B_n') -> Merge1/2
  If Action Subsystem3/1(Out1) -> Merge2/1
  If1/1 -> If Action Subsystem3/Action
  Relay1/1 -> Scope2/1, If1/1
  Relay/1 -> Scope3/1, If/1
  Abs/1 -> Scope3/2, Relay/1
  Q method/1(q_estimated) -> If Action Subsystem3/1(q_estimated), If Action Subsystem1/1(q_estimated)
  [flag] -> If Action Subsystem3/2(flag)
  Merge2/1 -> Out1/1, Unit Delay/1

== system CubeSatTEST/OBC/Navigation1/Sequential Rotations + Q method ==
  S_b : Inport
  Sn : Inport  Port=2
  B_b : Inport  Port=3
  Bn : Inport  Port=4
  alpha 1 : Inport  Port=5
  alpha 2 : Inport  Port=6
  Abs1 : Abs  SaturateOnIntegerOverflow=off
  If Action Subsystem1 : Subsystem  TreatAsAtomicUnit=on
  If1 : If  IfExpression=u1 < 0.2
  Merge : Merge
  Q method : Subsystem
      settings: PortSchema="{\"entries\":[{\"content\":{\"sides\":[{\"content\":{\"connectorIds\":[\"In1\",\"In2\",\"In3\",\"In4\"]},\"type\":\"ConnectorPlacement.EquallySpacedRectSide\",\"uuid\":\"15956c10-3c30-4cb4-a63c-f434daa5cd48\"},{\"content\":{\"connectorIds\":[\"Out1\"],\"side\":\"RIGHT\"},\"type\":\"ConnectorPlacement.EquallySpacedRectSide\",\"uuid\":\"3f26d307-35c8-43a0-9998-86e1286678fb\"},{\"content\":{\"connectorIds\":[\"In5\",\"In6\"],\"side\":\"TOP\"},\"type\":\"ConnectorPlacement.EquallySpacedRectSide\",\"uuid\":\"55f51305-766e-4e3f-8617-95c7676083b2\"}]},\"type\":\"ConnectorPlacement.EquallySpacedConnector\",\"uuid\":\"09b6cbb7-0430-4316-92af-7ec4423129aa\"}],\"packageUris\":[\"http://schema.mathworks.com/mf0/Connector/R2020b\"],\"version\":\"1.0\"}"
  Reference Rotator z : Subsystem
  Reference Rotator z1 : Subsystem
  Scope : Scope
  Selector1 : Selector  InputPortWidth=4  IndexOptions=Index vector (dialog)  Indices=4  OutputSizes=1
  Z : Subsystem  TreatAsAtomicUnit=on
  q_estimated : Outport
  wires:
  S_b/1 -> Z/3(S_b), Q method/1(S_b)
  B_b/1 -> Z/4(B_b), Q method/2(B_b)
  Selector1/1 -> Abs1/1
  [flag] -> Selector1/1
  Abs1/1 -> If1/1
  Sn/1 -> Z/7(S_n), Reference Rotator z1/1(S_N), Q method/3(S_N)
  Bn/1 -> Z/8(B_n), Reference Rotator z/1(S_N), Q method/4(B_N)
  Q method/1(q_estimated) -> If Action Subsystem1/1(q_estimated), [flag]
  If Action Subsystem1/1(Out1) -> Merge/1
  If1/1 -> If Action Subsystem1/Action
  If1/2 -> Z/Action
  Z/1(Out1) -> Merge/2
  Merge/1 -> Scope/1, q_estimated/1
  alpha 1/1 -> [alpha1]
  alpha 2/1 -> [alpha2]
  [alpha1] -> Q method/5(alpha 1)
  [alpha2] -> Q method/6(alpha 2)
  [alpha1] -> Z/1(q_estimated)
  [alpha2] -> Z/2(flag)
  Reference Rotator z1/1(Out1) -> Z/5(S_Nr)
  Reference Rotator z/1(B_N) -> Z/6(B_Nr)

== system CubeSatTEST/OBC/Navigation1/Sequential Rotations Playground ==
  Alpha1 : Inport
  Alpha2 : Inport  Port=2
  S_b : Inport  Port=3
  S_N : Inport  Port=4
  B_b : Inport  Port=5
  B_N : Inport  Port=6
  Constant : Constant  Value=[1; 1; 1; 1]
  Demux : Demux
  Enable second check : Subsystem  TreatAsAtomicUnit=on
  Enable second check1 : Subsystem  TreatAsAtomicUnit=on
  If : If  NumInputs=2  IfExpression=(u1 == 0)  ElseIfExpressions=(u2 == 0)
  If1 : If  NumInputs=3  IfExpression=(u1 == 1)&(u2==0)  ElseIfExpressions=(u1 == 1)&(u3==0)  ShowElse=off
  If2 : If  NumInputs=2  IfExpression=u1 == 0  ElseIfExpressions=u2 == 0
  If3 : If  NumInputs=3  IfExpression=(u1 == 1)&(u2==0)  ElseIfExpressions=(u1 == 1)&(u3==0)  ShowElse=off
  Max : Subsystem
  Max of Elements : MinMax  Function=max
  Memory : Memory  InitialCondition=[0;0;0;1]
  Merge : Merge  Inputs=4
  Merge1 : Merge  Inputs=4
  Product : Product
  Q method : Subsystem
      settings: PortSchema="{\"entries\":[{\"content\":{\"sides\":[{\"content\":{\"connectorIds\":[\"In1\",\"In2\",\"In3\",\"In4\"]},\"type\":\"ConnectorPlacement.EquallySpacedRectSide\",\"uuid\":\"15956c10-3c30-4cb4-a63c-f434daa5cd48\"},{\"content\":{\"connectorIds\":[\"Out1\"],\"side\":\"RIGHT\"},\"type\":\"ConnectorPlacement.EquallySpacedRectSide\",\"uuid\":\"3f26d307-35c8-43a0-9998-86e1286678fb\"},{\"content\":{\"connectorIds\":[\"In5\",\"In6\"],\"side\":\"TOP\"},\"type\":\"ConnectorPlacement.EquallySpacedRectSide\",\"uuid\":\"55f51305-766e-4e3f-8617-95c7676083b2\"}]},\"type\":\"ConnectorPlacement.EquallySpacedConnector\",\"uuid\":\"09b6cbb7-0430-4316-92af-7ec4423129aa\"}],\"packageUris\":[\"http://schema.mathworks.com/mf0/Connector/R2020b\"],\"version\":\"1.0\"}"
  Reference Rotator x : Subsystem
  Reference Rotator x1 : Subsystem
  Reference Rotator y : Subsystem
  Reference Rotator y1 : Subsystem
  Reference Rotator z : Subsystem
  Reference Rotator z1 : Subsystem
  Scope : Scope  NumInputPorts=3
  Scope1 : Scope
  Scope2 : Scope
  Subtract : Sum  Inputs=-+
  Switch Case Action Subsystem : Subsystem  TreatAsAtomicUnit=on
  Switch Case Action Subsystem1 : Subsystem  TreatAsAtomicUnit=on
  q_estimated : Outport
  wires:
  Alpha1/1 -> Q method/5(alpha 1)
  Alpha2/1 -> Q method/6(alpha 2)
  S_b/1 -> Q method/1(S_b)
  B_b/1 -> Q method/3(B_b)
  Switch Case Action Subsystem/1(Out1) -> Merge/1
  Reference Rotator x/1(Out1) -> Merge/2
  Reference Rotator y/1(Out1) -> Merge/3
  Reference Rotator z/1(Out1) -> Merge/4
  S_N/1 -> Reference Rotator x/1(S_N), Switch Case Action Subsystem/1(S_N), Reference Rotator y/1(S_N), Reference Rotator z/1(S_N)
  Reference Rotator x1/1(Out1) -> Merge1/2
  Reference Rotator y1/1(Out1) -> Merge1/3
  Switch Case Action Subsystem1/1(Out1) -> Merge1/1
  Reference Rotator z1/1(Out1) -> Merge1/4
  B_N/1 -> Reference Rotator z1/1(S_N), Reference Rotator y1/1(S_N), Reference Rotator x1/1(S_N), Switch Case Action Subsystem1/1(S_N)
  Merge1/1 -> Scope/3, Q method/4(B_N)
  Merge/1 -> Scope/2, Q method/2(S_N)
  Max/1(Index) -> Scope/1, Memory/1, q_estimated/1
  Memory/1 -> Scope2/1, [case]
  Q method/1(q_estimated) -> Scope1/1, Max/2(q)
  Max of Elements/1 -> Product/2
  Demux/1 -> If3/3, If1/3
  If/3 -> Enable second check/Action
  Product/1 -> Subtract/1
  If/1 -> Switch Case Action Subsystem/Action
  Demux/2 -> If1/2, If3/2
  Demux/4 -> If2/1, If/1
  Constant/1 -> Product/1
  Demux/3 -> If/2, If2/2
  If/2 -> Reference Rotator z/Action
  Enable second check/1(Out1) -> If1/1
  [case] -> Max/1(In1)
  If1/1 -> Reference Rotator y/Action
  If1/2 -> Reference Rotator x/Action
  If2/1 -> Switch Case Action Subsystem1/Action
  Enable second check1/1(Out1) -> If3/1
  If2/3 -> Enable second check1/Action
  If2/2 -> Reference Rotator z1/Action
  If3/1 -> Reference Rotator y1/Action
  If3/2 -> Reference Rotator x1/Action
  Subtract/1 -> Demux/1
  [case] -> Subtract/2, Max of Elements/1

== system CubeSatTEST/OBC/Normaliser (with Built In safety)/Norm1 ==
  Vector : Inport
  Add : Sum  Inputs=+++
  Demux : Demux  Outputs=3
  Sqrt : Sqrt
  Square : Math  Operator=square
  Square1 : Math  Operator=square
  Square2 : Math  Operator=square
  Norm : Outport
  wires:
  Square/1 -> Add/1
  Add/1 -> Sqrt/1
  Demux/3 -> Square1/1
  Square2/1 -> Add/2
  Square1/1 -> Add/3
  Demux/1 -> Square/1
  Demux/2 -> Square2/1
  Vector/1 -> Demux/1
  Sqrt/1 -> Norm/1

== system CubeSatTEST/OBC/Normaliser (with Built In safety)/Protected Division ==
  Vector : Inport
  Norm : Inport  Port=2
  Constant : Constant  Value=eps
  Divide : Product  Inputs=*/
  Switch : Switch  Criteria=u2 ~= 0  SaturateOnIntegerOverflow=off  InputSameDT=off
  Out1 : Outport
  wires:
  Divide/1 -> Out1/1
  Vector/1 -> Divide/1
  Norm/1 -> Switch/1, Switch/2
  Switch/1 -> Divide/2
  Constant/1 -> Switch/3

== system CubeSatTEST/OBC/Normaliser (with Built In safety)1/Norm1 ==
  Vector : Inport
  Add : Sum  Inputs=+++
  Demux : Demux  Outputs=3
  Sqrt : Sqrt
  Square : Math  Operator=square
  Square1 : Math  Operator=square
  Square2 : Math  Operator=square
  Norm : Outport
  wires:
  Square/1 -> Add/1
  Add/1 -> Sqrt/1
  Demux/3 -> Square1/1
  Square2/1 -> Add/2
  Square1/1 -> Add/3
  Demux/1 -> Square/1
  Demux/2 -> Square2/1
  Vector/1 -> Demux/1
  Sqrt/1 -> Norm/1

== system CubeSatTEST/OBC/Normaliser (with Built In safety)1/Protected Division ==
  Vector : Inport
  Norm : Inport  Port=2
  Constant : Constant  Value=eps
  Divide : Product  Inputs=*/
  Switch : Switch  Criteria=u2 ~= 0  SaturateOnIntegerOverflow=off  InputSameDT=off
  Out1 : Outport
  wires:
  Divide/1 -> Out1/1
  Vector/1 -> Divide/1
  Norm/1 -> Switch/1, Switch/2
  Switch/1 -> Divide/2
  Constant/1 -> Switch/3

== system CubeSatTEST/OBC/Reference/Conical Shadow Model ==
  note: Output Interface
  note: Input Interface
  note: Model is cylindrical shadow, formula was taken by Crassidis
  S_n : Inport
  r_n : Inport  Port=2
  Dot Product : DotProduct  OutDataTypeStr=Inherit: Inherit via internal rule
  Earth's Radius : Constant  Value=env.Earth.R
  Eclipse (1) : Subsystem  TreatAsAtomicUnit=on
  Gain : Gain  Gain=-1
  If : If  NumInputs=2  IfExpression=u1 < u2
  Merge : Merge
  Norm : Subsystem
  NotEclipse (0) : Subsystem  TreatAsAtomicUnit=on
  Sqrt : Sqrt
  Square : Math  Operator=square
  Square1 : Math  Operator=square
  Subtract : Sum  Inputs=+-
  eclipseFlag : Outport
  wires:
  r_n/1 -> Dot Product/2, Norm/1(Vector)  "r_n"
  S_n/1 -> Dot Product/1  "S_n"
  Norm/1(Norm) -> Square1/1  "norm_r"
  If/1 -> Eclipse (1)/Action
  If/2 -> NotEclipse (0)/Action
  Merge/1 -> eclipseFlag/1
  Eclipse (1)/1(One) -> Merge/1
  NotEclipse (0)/1(Zero) -> Merge/2
  Dot Product/1 -> If/1
  Gain/1 -> If/2
  Sqrt/1 -> Gain/1
  Subtract/1 -> Sqrt/1
  Square/1 -> Subtract/2
  Square1/1 -> Subtract/1
  Earth's Radius/1 -> Square/1  "earth_R"

== system CubeSatTEST/OBC/Reference/Kepler Integrator1 ==
  Add : Sum  Inputs=+-
  Add1 : Sum
  Add2 : Sum
  Clock : Clock
  Constant : Constant  Value=IC.theta
  Constant1 : Constant  Value=3/2
  Constant2 : Constant
  Constant3 : Constant  Value=2
  Constant4 : Constant  Value=orb.e
  Constant5 : Constant  Value=2
  Constant6 : Constant
  Constant7 : Constant  Value=IC.OM
  Constant8 : Constant  Value=2*pi
  Cosh : Trigonometry  Operator=cos
  Divide : Product  Inputs=*/
  Gain : Gain  Gain=orb.n
  Gain1 : Gain  Gain=orb.e
  Gain2 : Gain  Gain=orb.OMprec
  Integrator : Integrator  InitialConditionSource=external  WrapState=on  WrappedStateUpperValue=2*pi  WrappedStateLowerValue=0
  Mod : Math  Operator=mod
  Power : Math  Operator=pow
  Power1 : Math  Operator=pow
  Power2 : Math  Operator=pow
  th : Outport
  OM : Outport  Port=2
  wires:
  Constant/1 -> Integrator/2
  Integrator/1 -> Cosh/1, th/1
  Divide/1 -> Integrator/1
  Power/1 -> Divide/2
  Constant1/1 -> Power/2
  Constant2/1 -> Add/1
  Add/1 -> Power/1
  Power1/1 -> Add/2
  Constant3/1 -> Power1/2
  Constant4/1 -> Power1/1
  Gain/1 -> Divide/1
  Power2/1 -> Gain/1
  Constant5/1 -> Power2/2
  Add1/1 -> Power2/1
  Constant6/1 -> Add1/1
  Gain1/1 -> Add1/2
  Cosh/1 -> Gain1/1
  Constant7/1 -> Add2/2
  Gain2/1 -> Add2/1
  Clock/1 -> Gain2/1
  Add2/1 -> Mod/1
  Constant8/1 -> Mod/2
  Mod/1 -> OM/1
